simulink model "simuladorControlCuatrirrotor_summerschool_students"  (Simulink 8.5)
settings: Solver=ode45  StartTime=0.0  StopTime=720  FixedStep=0.06  MaxStep=0.06  RelTol=1e-3
values from neighbouring files (symbols this model uses):
  radio = 0.05    [simulaControl.m]
  ruta = [0,0;ruta]    [pintascdata.m]    (also in simulaControl.m = [4 10; 0 14; -4 10; 0 6; 6 10; 0 16; -6 10; 0 4; 8 10; 0 18])
libraries: simulink x5
settings Model: Creator=xblasco  LastModifiedBy=ramon
settings DebuggingCC: SolverPrmCheckMsg=warning  FcnCallInpInsideContextMsg=UseLocalSettings
settings SFSimCC: SimParseCustomCode=off

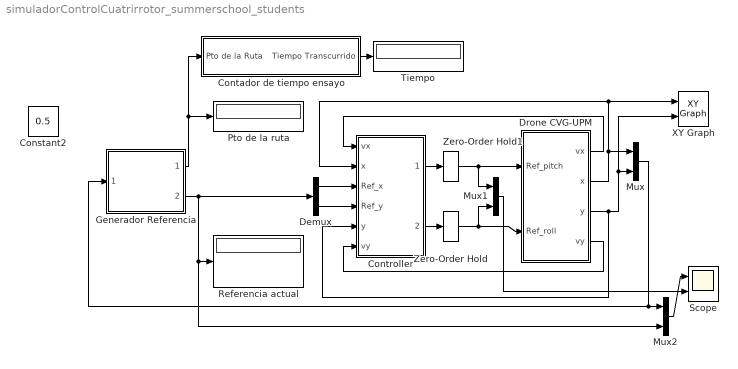
== system simuladorControlCuatrirrotor_summerschool_students ==
  Contador de tiempo ensayo : Subsystem
  Controller : Subsystem
  Demux : Demux  Outputs=2
  Drone CVG-UPM : Subsystem
      mask init:
      | % Old Icon code
      | % image(imread('Parrot_CEA.png'));
      | % port_label('input',1,'\fontsize{16}\bfRef pitch','texmode', 'on')
      | % port_label('input',2,'\fontsize{16}\bfRef roll','texmode', 'on')
      | % port_label('output',2,'\fontsize{16}\bfx','texmode', 'on')
      | % port_label('output',1,'\fontsize{16}\bfvx','texmode', 'on')
      | % port_label('output',3,'\fontsize{16}\bfy','texmode', 'on')
      | % port_label('output',4,'\fontsize{16}\bfvy','texmode', 'on')
  Generador Referencia : Subsystem
  Mux : Mux  Inputs=2
  Mux1 : Mux  Inputs=2
  Mux2 : Mux  Inputs=2
  Pto de la ruta : Display
  Referencia actual : Display
  Scope : Scope  NumInputPorts=2
      settings: YMin=-5~-1  YMax=15~1  SaveName=scdata  SampleInput=on  SampleTime=0.06
  Tiempo : Display
  XY Graph : simulink/Sinks/XY Graph  xmin=-20  xmax=20  ymin=-20  ymax=20  st=-1
  Zero-Order Hold : ZeroOrderHold  SampleTime=0.06
  Zero-Order Hold1 : ZeroOrderHold  SampleTime=0.06
  Constant2 : Constant  IOType=siggen  Value=0.5
  wires:
  Generador Referencia/2(Siguiente pos) -> Referencia actual/1, Mux2/2, Demux/1
  Generador Referencia/1(Pto de la ruta) -> Pto de la ruta/1, Contador de tiempo ensayo/1(Pto de la Ruta)
  Controller/1(Ref_Pitch) -> Zero-Order Hold1/1
  Controller/2(Ref_Roll) -> Zero-Order Hold/1
  Mux/1 -> Generador Referencia/1(Posicion  actual), Mux2/1
  Zero-Order Hold/1 -> Mux1/2, Drone CVG-UPM/2(Ref_roll)
  Zero-Order Hold1/1 -> Mux1/1, Drone CVG-UPM/1(Ref_pitch)
  Drone CVG-UPM/2(x) -> Mux/1, Controller/2(x), XY Graph/1
  Drone CVG-UPM/3(y) -> Controller/5(y), XY Graph/2, Mux/2
  Mux1/1 -> Scope/2
  Drone CVG-UPM/1(vx) -> Controller/1(vx)
  Mux2/1 -> Scope/1
  Contador de tiempo ensayo/1(Tiempo Transcurrido) -> Tiempo/1
  Drone CVG-UPM/4(vy) -> Controller/6(vy)
  Demux/1 -> Controller/3(Ref_x)
  Demux/2 -> Controller/4(Ref_y)

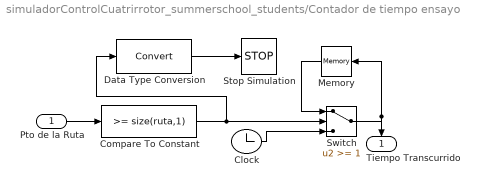
== system simuladorControlCuatrirrotor_summerschool_students/Contador de tiempo ensayo ==
  Pto de la Ruta : Inport
  Clock : Clock
  Compare To Constant : simulink/Logic and Bit Operations/Compare To Constant  relop=>=  const=size(ruta,1)  OutDataTypeStr=uint8
  Data Type Conversion : DataTypeConversion
  Memory : Memory
  Stop Simulation : Stop
  Switch : Switch  Threshold=1
  Tiempo Transcurrido : Outport
  wires:
  Clock/1 -> Switch/3
  Compare To Constant/1 -> Switch/2, Data Type Conversion/1
  Switch/1 -> Memory/1, Tiempo Transcurrido/1
  Memory/1 -> Switch/1
  Data Type Conversion/1 -> Stop Simulation/1
  Pto de la Ruta/1 -> Compare To Constant/1

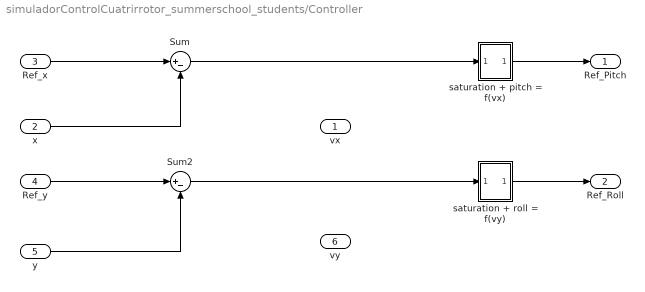
== system simuladorControlCuatrirrotor_summerschool_students/Controller ==
  vx : Inport
  x : Inport  Port=2
  Ref_x : Inport  Port=3
  Ref_y : Inport  Port=4
  y : Inport  Port=5
  vy : Inport  Port=6
  Sum : Sum  Inputs=|+-
  Sum2 : Sum  Inputs=|+-
  saturation + pitch = f(vx) : Subsystem
      mask Display:
      | u = -3:0.2:3;
      | plot(u,-asin(u./3.572)/2.541);
      | plot(u,zeros(length(u),1));
      | plot([0 0],[-.4 .4]);
  saturation + roll = f(vy) : Subsystem
      mask Display:
      | u = -1.8:0.1:1.8;
      | plot(u,asin(u/3.151)/2.094);
      | plot(u,zeros(length(u),1));
      | plot([0 0],[-.3 .3]);
  Ref_Pitch : Outport
  Ref_Roll : Outport  Port=2
  wires:
  Ref_x/1 -> Sum/1
  Ref_y/1 -> Sum2/1
  x/1 -> Sum/2
  y/1 -> Sum2/2
  saturation + pitch = f(vx)/1(pitch) -> Ref_Pitch/1
  saturation + roll = f(vy)/1(roll) -> Ref_Roll/1
  Sum2/1 -> saturation + roll = f(vy)/1(vy)
  Sum/1 -> saturation + pitch = f(vx)/1(vx)

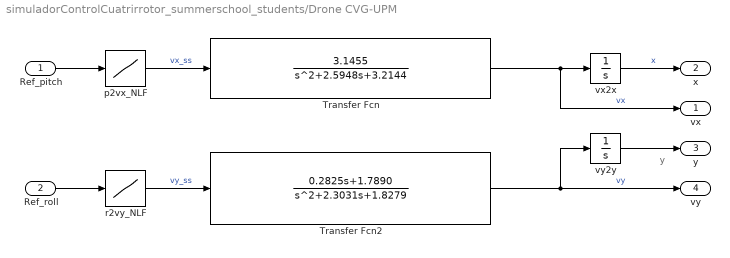
== system simuladorControlCuatrirrotor_summerschool_students/Drone CVG-UPM ==
  note: y
  Ref_pitch : Inport
  Ref_roll : Inport  Port=2
  Transfer Fcn : TransferFcn  Numerator=[3.1455]  Denominator="[ 1.0000    2.5948    3.2144]"
  Transfer Fcn2 : TransferFcn  Numerator="[0.2825    1.7890]"  Denominator="[1.0000    2.3031    1.8279]"
  p2vx_NLF : Lookup  InputValues=|  Table=|
      InputValues=|
      | [-1
      | -0.899999999999999
      | -0.799999999999999
      | -0.700000000000001
      | -0.600000000000001
      | -0.554327720000000
      | -0.487624560000000
      | -0.408038037500000
      | -0.362068970000000
      | -0.333010170000000
      | -0.299309153333334
      | -0.254820010000000
      | -0.231935350000000
      | -0.195105166666667
      | -0.160945750000000
      | -0.111971006666667
      | -0.0798540220000001
      | 0
      | 0.0798540220000001
      | 0.111971006666667
      | 0.160945750000000
      | 0.195105166666667
      | 0.231935350000000
      | 0.254820010000000
      | 0.299309153333334
      | 0.333010170000000
      | 0.362068970000000
      | 0.412860860000000
      | 0.487624560000000
      | 0.554327720000000
      | 0.600000000000001
      | 0.700000000000001
      | 0.799999999999999
      | 0.899999999999999
      | 1
      | ]
      Table=|
      | [2.94150928615385
      | 3.04525285846154
      | 3.00999432153846
      | 3.26915892153846
      | 3.32566329384615
      | 3.21536306865672
      | 3.04352811060084
      | 2.98373075134615
      | 2.87725081194030
      | 2.72743332761194
      | 2.52254295732874
      | 2.17497777985075
      | 1.98995770037313
      | 1.67598362847302
      | 1.38764086716418
      | 0.979314068412553
      | 0.619557218208955
      | 0
      | -0.634548146865672
      | -0.972497305634902
      | -1.39010210970149
      | -1.67803360287792
      | -1.98244432201493
      | -2.15552099328358
      | -2.51882706779181
      | -2.74484146641791
      | -2.87231153059701
      | -2.99661401608266
      | -3.03228925497130
      | -3.22903016567164
      | -3.33884447692308
      | -3.27388889384615
      | -3.01520380307692
      | -3.09037704153846
      | -2.90956140769231
      | ]
  r2vy_NLF : Lookup  InputValues=|  Table=|
      InputValues=|
      | [-1
      | -0.899999999999999
      | -0.799999999999999
      | -0.700000000000001
      | -0.600000000000001
      | -0.554327720000000
      | -0.500000000000000
      | -0.465116950000000
      | -0.424264070000000
      | -0.400000000000000
      | -0.375365390000000
      | -0.362068970000000
      | -0.299309153333334
      | -0.284772200000000
      | -0.231935350000000
      | -0.196880932000000
      | -0.167681415000000
      | -0.137937330000000
      | -0.103699940000000
      | 0
      | 0.103699940000000
      | 0.137937330000000
      | 0.167681415000000
      | 0.196880932000000
      | 0.231935350000000
      | 0.284772200000000
      | 0.299309153333334
      | 0.362068970000000
      | 0.375365390000000
      | 0.400000000000000
      | 0.424264070000000
      | 0.465116950000000
      | 0.500000000000000
      | 0.554327720000000
      | 0.600000000000001
      | 0.700000000000001
      | 0.799999999999999
      | 0.899999999999999
      | 1
      | ]
      Table=|
      | [-1.90950885076923
      | -2.17042302769231
      | -2.08382318000000
      | -2.12906611538462
      | -2.11523329538462
      | -2.01770647985075
      | -1.89077186615385
      | -1.76205706044776
      | -1.61365458358209
      | -1.50208098615385
      | -1.43325184104478
      | -1.37513765373134
      | -1.73740862189820
      | -1.81467803432836
      | -1.49700599291045
      | -1.26829053070034
      | -1.07653842145522
      | -0.897240183731343
      | -0.639549895111366
      | 0
      | 0.654743088496747
      | 0.879614668582090
      | 1.07783751735075
      | 1.26734386833525
      | 1.48971678843284
      | 1.82527751492537
      | 1.73787658138538
      | 1.38022974029851
      | 1.42903529029851
      | 1.51989753538462
      | 1.60039535000000
      | 1.75354396194030
      | 1.89258457692308
      | 2.03288599850746
      | 2.10148282769231
      | 2.12578287384615
      | 2.06483130000000
      | 2.15472636461539
      | 1.89130308000000
      | ]
  vx2x : Integrator
  vy2y : Integrator
  vx : Outport
  x : Outport  Port=2
  y : Outport  Port=3
  vy : Outport  Port=4
  wires:
  Transfer Fcn/1 -> vx/1, vx2x/1  "vx"
  r2vy_NLF/1 -> Transfer Fcn2/1  "vy_ss"
  p2vx_NLF/1 -> Transfer Fcn/1  "vx_ss"
  Ref_roll/1 -> r2vy_NLF/1
  vx2x/1 -> x/1  "x"
  vy2y/1 -> y/1
  Transfer Fcn2/1 -> vy/1, vy2y/1  "vy"
  Ref_pitch/1 -> p2vx_NLF/1

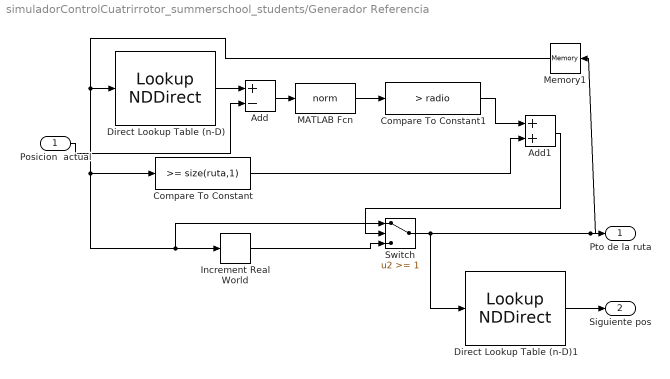
== system simuladorControlCuatrirrotor_summerschool_students/Generador Referencia ==
  Posicion  actual : Inport  PortDimensions=2
  Add : Sum  Inputs=+-
  Add1 : Sum
  Compare To Constant : simulink/Logic and Bit Operations/Compare To Constant  relop=>=  const=size(ruta,1)  OutDataTypeStr=uint8
  Compare To Constant1 : simulink/Logic and Bit Operations/Compare To Constant  relop=>  const=radio  OutDataTypeStr=uint8
  Direct Lookup Table (n-D) : LookupNDDirect  InputsSelectThisObjectFromTable=Column  Table=ruta'
  Direct Lookup Table (n-D)1 : LookupNDDirect  InputsSelectThisObjectFromTable=Column  Table=ruta'
  Increment Real World : simulink/Additional Math & Discrete/Additional Math: Increment - Decrement/Increment Real World
  MATLAB Fcn : MATLABFcn  MATLABFcn=norm  Output1D=off
  Memory1 : Memory
  Switch : Switch  Threshold=1
  Pto de la ruta : Outport
  Siguiente pos : Outport  Port=2
  wires:
  Direct Lookup Table (n-D)/1 -> Add/1
  Add/1 -> MATLAB Fcn/1
  Increment Real World/1 -> Switch/3
  Switch/1 -> Direct Lookup Table (n-D)1/1, Pto de la ruta/1, Memory1/1
  Posicion  actual/1 -> Add/2
  Direct Lookup Table (n-D)1/1 -> Siguiente pos/1
  MATLAB Fcn/1 -> Compare To Constant1/1
  Compare To Constant1/1 -> Add1/1
  Compare To Constant/1 -> Add1/2
  Add1/1 -> Switch/2
  Memory1/1 -> Direct Lookup Table (n-D)/1, Switch/1, Increment Real World/1, Compare To Constant/1

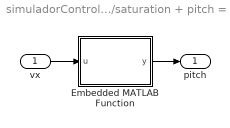
== system simuladorControlCuatrirrotor_summerschool_students/Controller/saturation + pitch = f(vx) ==
  vx : Inport
  Embedded MATLAB Function : MATLAB Function  TreatAsAtomicUnit=on
  pitch : Outport
  wires:
  vx/1 -> Embedded MATLAB Function/1(u)
  Embedded MATLAB Function/1(y) -> pitch/1

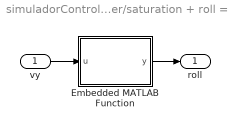
== system simuladorControlCuatrirrotor_summerschool_students/Controller/saturation + roll = f(vy) ==
  vy : Inport
  Embedded MATLAB Function : MATLAB Function  TreatAsAtomicUnit=on
  roll : Outport
  wires:
  vy/1 -> Embedded MATLAB Function/1(u)
  Embedded MATLAB Function/1(y) -> roll/1

== matlab function Controller/saturation + pitch = f(vx)/Embedded MATLAB Function ==
  data: u input double; y output double
function y = fcn(u)
%#eml

% Codigo 1:
% ---------

% usup =  3;
% uinf = -3;
% 
% if (u > usup)
%     u = usup;
% else if (u < uinf)
%         u = uinf;
%     end
% end
% 
% y = -asin(u/3.572)/2.541;



% Codigo 2:
% ---------

usup =  3.33;
uinf = -3.33;

if (u > usup)
    u = usup;
else if (u < uinf)
        u = uinf;
    end
end

if (-3 <= u) && (u <= 3)
    y = -asin(u/3.572)/2.541;
else 
     aux = abs(u);
     vx1 = 3;
     vx2 = 3.33;
     p1 =  0.4876;
     p2 =  .6;
     y = -sign(u) * (p1 + (aux - vx1)*(p2-p1)/(vx2-vx1));
end

== matlab function Controller/saturation + roll = f(vy)/Embedded MATLAB Function ==
  data: u input double; y output double
function y = fcn(u)
%#eml


% % Codigo 1:
% % ---------
% 
% usup =  1.8;
% uinf = -1.8;
% 
% if (u > usup)
%     u = usup;
% else if (u < uinf)
%         u = uinf;
%     end
% end
% 
% y = asin(u(1)/3.151)/2.094;



% Codigo 2:
% ---------

usup =  2.1;
uinf = -2.1;

if (u > usup)
    u = usup;
else if (u < uinf)
        u = uinf;
    end
end

if (-1.8 <= u) && (u <= 1.8)
    y = asin(u(1)/3.151)/2.094;
else 
     aux = abs(u);
     vy1 = 1.8;
     vy2 = 2.1;
     r1 =  0.48;
     r2 =  .6;
     y = sign(u) * (r1 + (aux - vy1)*(r2-r1)/(vy2-vy1));
end
